simulink model "receive_a825_r2016b"  (R2016b)
settings: Solver=VariableStepAuto  StartTime=0.0  StopTime=10.0  RelTol=1e-3
model workspace (MAT data in the model file):
  ED247Configuration(1).name = 'Stream0'
  ED247Configuration(1).direction = 'IN'
  ED247Configuration(1).type = 'uint8'
  ED247Configuration(1).dimensions = 1
  ED247Configuration(1).width = 3
  ED247Configuration(1).size = 3
  ED247Configuration(1).sample_time = 1
  ED247Configuration(1).validity_duration = 1
  ED247Configuration(1).signal_type = 'A825'
  ED247Configuration(1).sample_size = 3
  ED247Configuration(2).name = 'Stream1'
  ED247Configuration(2).direction = 'IN'
  ED247Configuration(2).type = 'uint8'
  ED247Configuration(2).dimensions = 1
  ED247Configuration(2).width = 5
  ED247Configuration(2).size = 5
  ED247Configuration(2).sample_time = 0.0640000030398
  ED247Configuration(2).validity_duration = 0.0640000030398
  ED247Configuration(2).signal_type = 'A825'
  ED247Configuration(2).sample_size = 5
  ED247Configuration(3).name = 'Stream0'
  ED247Configuration(3).direction = 'OUT'
  ED247Configuration(3).type = 'uint8'
  ED247Configuration(3).dimensions = 1
  ED247Configuration(3).width = 3
  ED247Configuration(3).size = 3
  ED247Configuration(3).sample_time = 1
  ED247Configuration(3).validity_duration = 1
  ED247Configuration(3).signal_type = 'A825'
  ED247Configuration(3).sample_size = 3
  ED247Configuration(4).name = 'Stream1'
  ED247Configuration(4).direction = 'OUT'
  ED247Configuration(4).type = 'uint8'
  ED247Configuration(4).dimensions = 1
  ED247Configuration(4).width = 5
  ED247Configuration(4).size = 5
  ED247Configuration(4).sample_time = 0.0640000030398
  ED247Configuration(4).validity_duration = 0.0640000030398
  ED247Configuration(4).signal_type = 'A825'
  ED247Configuration(4).sample_size = 5
libraries: lib_ed247 x2
settings Model: Creator=odufour  LastModifiedBy=odufour
settings DataIOCC: ReturnWorkspaceOutputs=on
settings DebuggingCC: InheritedTsInSrcMsg=none
settings SFSimCC: SimUseLocalCustomCode=on
settings RTWCC: RTWUseLocalCustomCode=on

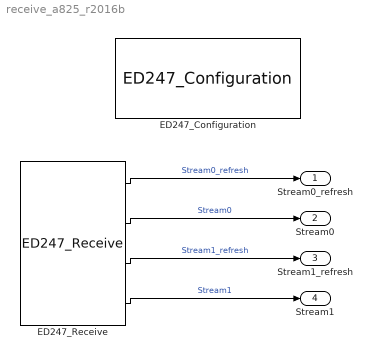
== system receive_a825_r2016b ==
  ED247_Configuration : lib_ed247/ED247_Configuration  configurationFilename='ecic_func_exchange_a825_uc_tester.xml'  enableLog=off  logFilename=''
  ED247_Receive : lib_ed247/ED247_Receive  enable_refresh=on  refresh_factor=1  sample_time=-1  show_port_labels=on
  Stream0_refresh : Outport
  Stream0 : Outport  Port=2  OutDataTypeStr=uint8  PortDimensions=3  SampleTime=0.1
  Stream1_refresh : Outport  Port=3
  Stream1 : Outport  Port=4  OutDataTypeStr=uint8  PortDimensions=5  SampleTime=0.1
  wires:
  ED247_Receive/2 -> Stream0/1  "Stream0"
  ED247_Receive/4 -> Stream1/1  "Stream1"
  ED247_Receive/1 -> Stream0_refresh/1  "Stream0_refresh"
  ED247_Receive/3 -> Stream1_refresh/1  "Stream1_refresh"
